simulink model "Simulator_Reduced"  (R2023a)
settings: Solver=ode4  StartTime=0.0  StopTime=Parameters.Simulink.sim_time_s  FixedStep=Parameters.Simulink.time_step_s  RelTol=1e-3
undefined symbols (not defined in the file): Parameters
libraries: eeGeneralControl x1
settings Model: Creator=thesa  LastModifiedBy=thesa
settings OptimizationCC: SimCompilerOptimization=on  AccelVerboseBuild=on
settings ModelReferenceCC: EnableParallelModelReferenceBuilds=on

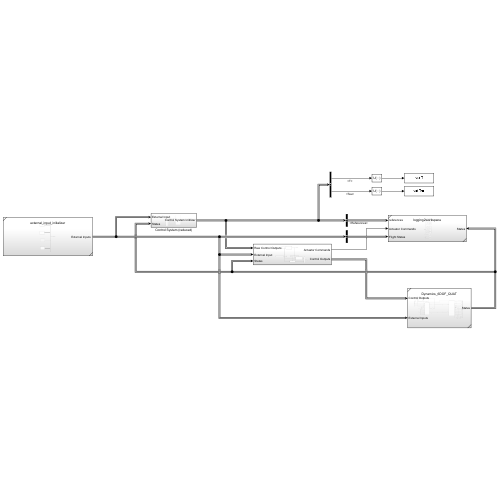
[thumbnail: Simulink's stored preview of the top-level diagram]
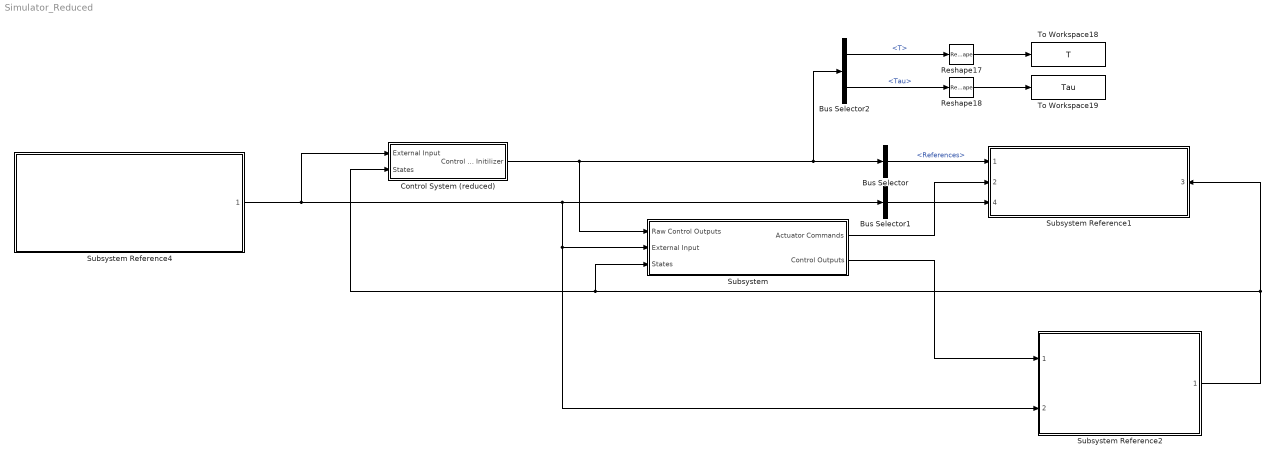
== system Simulator_Reduced ==
  Bus Selector : BusSelector  OutputSignals=References
  Bus Selector1 : BusSelector  OutputSignals=Pilot Input.ARMED,Pilot Input.FLIGHT_MODE  OutputAsBus=on
  Bus Selector2 : BusSelector  OutputSignals=Control Outputs.T,Control Outputs.Tau
  Control System (reduced) : Subsystem
  Reshape17 : Reshape
  Reshape18 : Reshape
  Subsystem : Subsystem
  Subsystem Reference1 : Subsystem  ReferencedSubsystem=logging2workspace
      settings: PortSchema="{\"entries\":[{\"content\":{\"sides\":[{\"content\":{\"connectorIds\":[\"In1\",\"In2\",\"In4\"]},\"type\":\"ConnectorPlacement.EquallySpacedRectSide\",\"uuid\":\"9edd3e15-5130-45dd-9916-21c08d031682\"},{\"content\":{\"connectorIds\":[\"In3\"],\"side\":\"RIGHT\"},\"type\":\"ConnectorPlacement.EquallySpacedRectSide\",\"uuid\":\"954423d3-db16-40ed-81b7-a6b5cde1e64c\"},{\"content\":{\"side\":\"TOP\"},\"type\":\"ConnectorPlacement.EquallySpacedRectSide\",\"uuid\":\"3251a3bf-10b0-45d6-866e-917fc661c50a\"}]},\"type\":\"ConnectorPlacement.EquallySpacedConnector\",\"uuid\":\"39e626d0-b0bd-4592-9fe5-df80528652ac\"}],\"packageUris\":[\"http://schema.mathworks.com/mf0/Connector/R2020b\"],\"version\":\"1.0\"}"
  Subsystem Reference2 : Subsystem  ReferencedSubsystem=Dynamics_6DOF_QUAT
  Subsystem Reference4 : Subsystem  ReferencedSubsystem=external_input_initializer
  To Workspace18 : ToWorkspace  VariableName=T  SampleTime=-1
  To Workspace19 : ToWorkspace  VariableName=Tau  SampleTime=-1
  wires:
  Subsystem Reference4/1 -> Bus Selector1/1, Subsystem Reference2/2, Subsystem/2(External Input), Control System (reduced)/1(External Input)
  Bus Selector/1 -> Subsystem Reference1/1  "<References>"
  Bus Selector1/1 -> Subsystem Reference1/4
  Control System (reduced)/1(Control System Initilizer) -> Subsystem/1(Raw Control Outputs), Bus Selector2/1, Bus Selector/1
  Reshape17/1 -> To Workspace18/1
  Reshape18/1 -> To Workspace19/1
  Bus Selector2/2 -> Reshape18/1  "<Tau>"
  Bus Selector2/1 -> Reshape17/1  "<T>"
  Subsystem/1(Actuator Commands) -> Subsystem Reference1/2
  Subsystem/2(Control Outputs) -> Subsystem Reference2/1
  Subsystem Reference2/1 -> Subsystem/3(States), Control System (reduced)/2(States), Subsystem Reference1/3

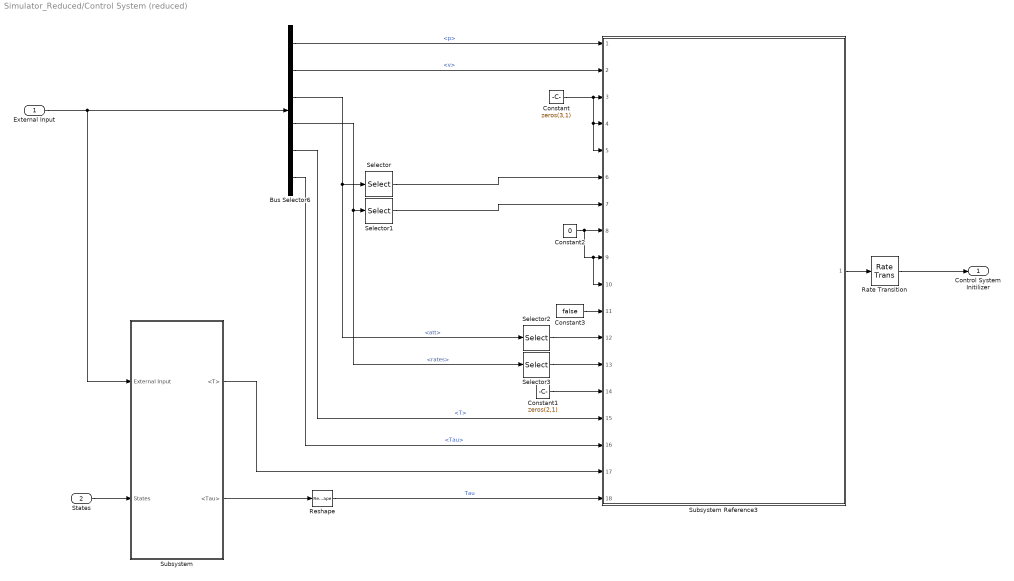
== system Simulator_Reduced/Control System (reduced) ==
  External Input : Inport
  States : Inport  Port=2
  Bus Selector6 : BusSelector  OutputSignals=Control Gains.K_matrix_control.ref.p,Control Gains.K_matrix_control.ref.v,Control Gains.K_matrix_control.ref.att,Control Gains.K_matrix_control.ref.rates,Control Gains.K_matrix_control.ref.T,Control Gains.K_matrix_control.ref.Tau
  Constant : Constant  Value=zeros(3,1)
  Constant1 : Constant  Value=zeros(2,1)
  Constant2 : Constant  Value=0
  Constant3 : Constant  Value=false
  Rate Transition : RateTransition  OutPortSampleTimeOpt=Inherit
  Reshape : Reshape  OutputDimensionality=Column vector (2-D)
  Selector : Selector  InputPortWidth=3  IndexOptions=Index vector (dialog)  Indices=[3]  OutputSizes=1
  Selector1 : Selector  InputPortWidth=3  IndexOptions=Index vector (dialog)  Indices=[3]  OutputSizes=1
  Selector2 : Selector  InputPortWidth=3  IndexOptions=Index vector (dialog)  Indices=[1,2]  OutputSizes=1
  Selector3 : Selector  InputPortWidth=3  IndexOptions=Index vector (dialog)  Indices=[1,2]  OutputSizes=1
  Subsystem : Subsystem
  Subsystem Reference3 : Subsystem  ReferencedSubsystem=control_initializer
  Control System Initilizer : Outport
  wires:
  Bus Selector6/3 -> Selector2/1, Selector/1  "<att>"
  External Input/1 -> Bus Selector6/1, Subsystem/1(External Input)
  Reshape/1 -> Subsystem Reference3/18  "Tau"
  Constant2/1 -> Subsystem Reference3/10, Subsystem Reference3/9, Subsystem Reference3/8
  Bus Selector6/4 -> Selector3/1, Selector1/1  "<rates>"
  Subsystem Reference3/1 -> Rate Transition/1
  Bus Selector6/1 -> Subsystem Reference3/1  "<p>"
  Bus Selector6/2 -> Subsystem Reference3/2  "<v>"
  Constant/1 -> Subsystem Reference3/5, Subsystem Reference3/4, Subsystem Reference3/3
  Selector/1 -> Subsystem Reference3/6
  Selector1/1 -> Subsystem Reference3/7
  Constant3/1 -> Subsystem Reference3/11
  Selector2/1 -> Subsystem Reference3/12
  Selector3/1 -> Subsystem Reference3/13
  Constant1/1 -> Subsystem Reference3/14
  Bus Selector6/5 -> Subsystem Reference3/15  "<T>"
  Bus Selector6/6 -> Subsystem Reference3/16  "<Tau>"
  Rate Transition/1 -> Control System Initilizer/1
  States/1 -> Subsystem/2(States)
  Subsystem/1(<T>) -> Subsystem Reference3/17
  Subsystem/2(<Tau>) -> Reshape/1

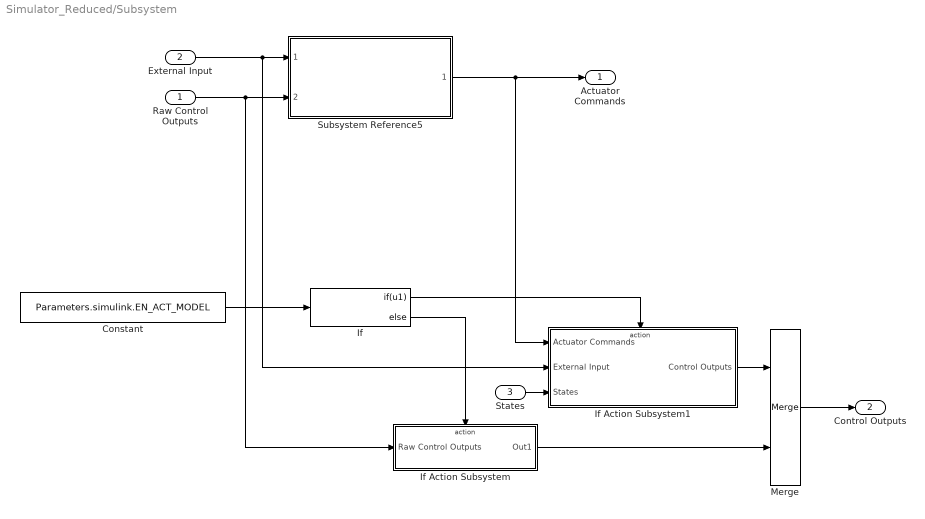
== system Simulator_Reduced/Subsystem ==
  Raw Control Outputs : Inport
  External Input : Inport  Port=2
  States : Inport  Port=3
  Constant : Constant  Value=Parameters.simulink.EN_ACT_MODEL
  If : If  IfExpression=u1
  If Action Subsystem : Subsystem  TreatAsAtomicUnit=on
  If Action Subsystem1 : Subsystem  TreatAsAtomicUnit=on
  Merge : Merge
  Subsystem Reference5 : Subsystem  ReferencedSubsystem=mixer
  Actuator Commands : Outport
  Control Outputs : Outport  Port=2
  wires:
  Subsystem Reference5/1 -> If Action Subsystem1/1(Actuator Commands), Actuator Commands/1
  Merge/1 -> Control Outputs/1
  External Input/1 -> If Action Subsystem1/2(External Input), Subsystem Reference5/1
  Raw Control Outputs/1 -> Subsystem Reference5/2, If Action Subsystem/1(Raw Control Outputs)
  If/1 -> If Action Subsystem1/Action
  If/2 -> If Action Subsystem/Action
  Constant/1 -> If/1
  If Action Subsystem1/1(Control Outputs) -> Merge/1
  If Action Subsystem/1(Out1) -> Merge/2
  States/1 -> If Action Subsystem1/3(States)

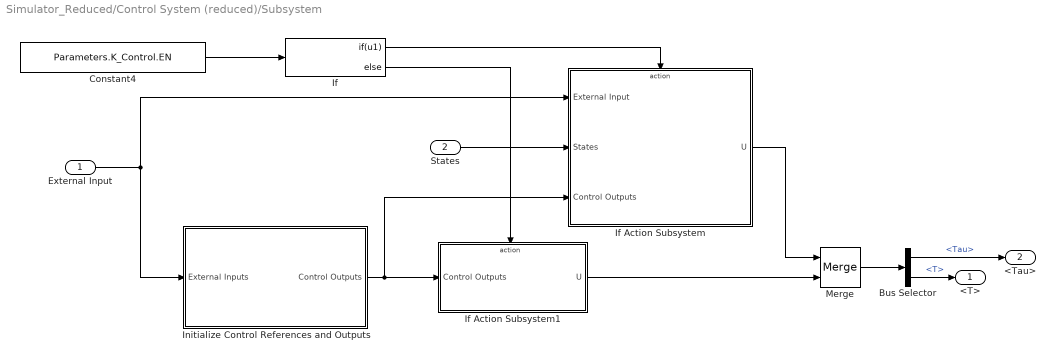
== system Simulator_Reduced/Control System (reduced)/Subsystem ==
  External Input : Inport
  States : Inport  Port=2
  Bus Selector : BusSelector  OutputSignals=Tau,T
  Constant4 : Constant  Value=Parameters.K_Control.EN
  If : If  IfExpression=u1
  If Action Subsystem : Subsystem  TreatAsAtomicUnit=on
  If Action Subsystem1 : Subsystem  TreatAsAtomicUnit=on
  Initialize Control References and Outputs : Subsystem
  Merge : Merge
  <T> : Outport
  <Tau> : Outport  Port=2
  wires:
  If/1 -> If Action Subsystem/Action
  Merge/1 -> Bus Selector/1
  If Action Subsystem/1(U) -> Merge/1
  If Action Subsystem1/1(U) -> Merge/2
  If/2 -> If Action Subsystem1/Action
  External Input/1 -> Initialize Control References and Outputs/1(External Inputs), If Action Subsystem/1(External Input)
  Constant4/1 -> If/1
  States/1 -> If Action Subsystem/2(States)
  Bus Selector/2 -> <T>/1  "<T>"
  Bus Selector/1 -> <Tau>/1  "<Tau>"
  Initialize Control References and Outputs/1(Control Outputs) -> If Action Subsystem/3(Control Outputs), If Action Subsystem1/1(Control Outputs)

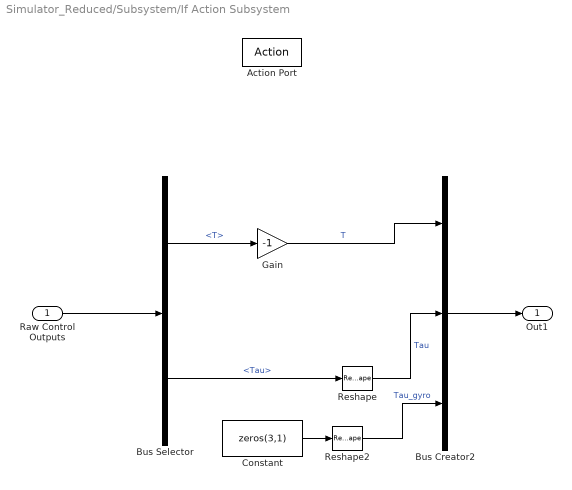
== system Simulator_Reduced/Subsystem/If Action Subsystem ==
  Raw Control Outputs : Inport
  Action Port : ActionPort  InitializeStates=reset  ActionPortLabel=else
  Bus Creator2 : BusCreator  Inputs=3
  Bus Selector : BusSelector  OutputSignals=Control Outputs.T,Control Outputs.Tau
  Constant : Constant  Value=zeros(3,1)
  Gain : Gain  Gain=-1
  Reshape : Reshape  OutputDimensionality=Column vector (2-D)
  Reshape2 : Reshape  OutputDimensionality=Column vector (2-D)
  Out1 : Outport
  wires:
  Bus Creator2/1 -> Out1/1
  Reshape/1 -> Bus Creator2/2  "Tau"
  Bus Selector/2 -> Reshape/1  "<Tau>"
  Bus Selector/1 -> Gain/1  "<T>"
  Raw Control Outputs/1 -> Bus Selector/1
  Gain/1 -> Bus Creator2/1  "T"
  Reshape2/1 -> Bus Creator2/3  "Tau_gyro"
  Constant/1 -> Reshape2/1

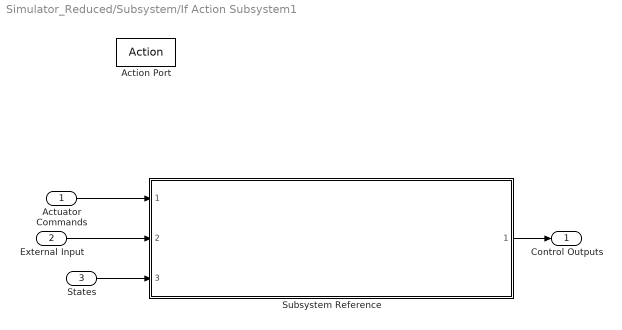
== system Simulator_Reduced/Subsystem/If Action Subsystem1 ==
  Actuator Commands : Inport
  External Input : Inport  Port=2
  States : Inport  Port=3
  Action Port : ActionPort  InitializeStates=reset  ActionPortLabel=if(u1)
  Subsystem Reference : Subsystem  ReferencedSubsystem=cmds2forces_map
  Control Outputs : Outport
  wires:
  Subsystem Reference/1 -> Control Outputs/1
  External Input/1 -> Subsystem Reference/2
  Actuator Commands/1 -> Subsystem Reference/1
  States/1 -> Subsystem Reference/3

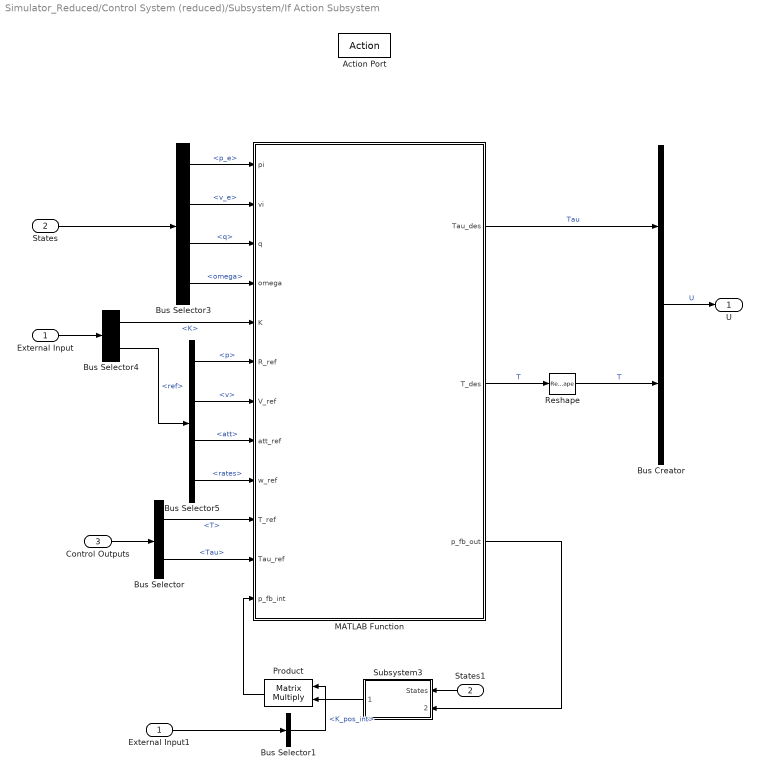
== system Simulator_Reduced/Control System (reduced)/Subsystem/If Action Subsystem ==
  External Input : Inport
  States : Inport  Port=2
  Control Outputs : Inport  Port=3
  Action Port : ActionPort  InitializeStates=reset  ActionPortLabel=if(u1)
  Bus Creator : BusCreator  Inputs=2
  Bus Selector : BusSelector  OutputSignals=T,Tau
  Bus Selector1 : BusSelector  OutputSignals=Control Gains.K_matrix_control.K_pos_int
  Bus Selector3 : BusSelector  OutputSignals=p_e,v_e,q,omega
  Bus Selector4 : BusSelector  OutputSignals=Control Gains.K_matrix_control.K,Control Gains.K_matrix_control.ref
  Bus Selector5 : BusSelector  OutputSignals=p,v,att,rates
  External Input1 : InportShadow
  MATLAB Function : MATLAB Function  TreatAsAtomicUnit=on
  Product : Product  Multiplication=Matrix(*)
  Reshape : Reshape  OutputDimensionality=Column vector (2-D)
  States1 : InportShadow  Port=2
  Subsystem3 : Subsystem
  U : Outport
  wires:
  Bus Selector5/4 -> MATLAB Function/9(w_ref)  "<rates>"
  MATLAB Function/2(T_des) -> Reshape/1  "T"
  Bus Selector4/2 -> Bus Selector5/1  "<ref>"
  Bus Selector3/2 -> MATLAB Function/2(vi)  "<v_e>"
  Bus Selector4/1 -> MATLAB Function/5(K)  "<K>"
  MATLAB Function/1(Tau_des) -> Bus Creator/1  "Tau"
  Bus Selector3/1 -> MATLAB Function/1(pi)  "<p_e>"
  Bus Selector3/3 -> MATLAB Function/3(q)  "<q>"
  States/1 -> Bus Selector3/1
  Bus Selector3/4 -> MATLAB Function/4(omega)  "<omega>"
  Bus Selector5/3 -> MATLAB Function/8(att_ref)  "<att>"
  Bus Selector5/2 -> MATLAB Function/7(V_ref)  "<v>"
  External Input/1 -> Bus Selector4/1
  Bus Selector5/1 -> MATLAB Function/6(R_ref)  "<p>"
  Reshape/1 -> Bus Creator/2  "T"
  Bus Creator/1 -> U/1  "U"
  External Input1/1 -> Bus Selector1/1
  Product/1 -> MATLAB Function/12(p_fb_int)
  Bus Selector1/1 -> Product/1  "<K_pos_int>"
  Subsystem3/1(p_fb_int) -> Product/2
  MATLAB Function/3(p_fb_out) -> Subsystem3/2(p_fb_out)
  States1/1 -> Subsystem3/1(States)
  Control Outputs/1 -> Bus Selector/1
  Bus Selector/1 -> MATLAB Function/10(T_ref)  "<T>"
  Bus Selector/2 -> MATLAB Function/11(Tau_ref)  "<Tau>"

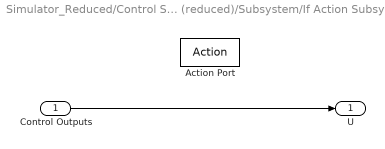
== system Simulator_Reduced/Control System (reduced)/Subsystem/If Action Subsystem1 ==
  Control Outputs : Inport
  Action Port : ActionPort  ActionPortLabel=else
  U : Outport
  wires:
  Control Outputs/1 -> U/1

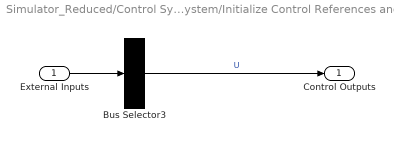
== system Simulator_Reduced/Control System (reduced)/Subsystem/Initialize Control References and Outputs ==
  External Inputs : Inport
  Bus Selector3 : BusSelector  OutputSignals=Control Gains.K_matrix_control.ref.Tau,Control Gains.K_matrix_control.ref.T  OutputAsBus=on
  Control Outputs : Outport
  wires:
  Bus Selector3/1 -> Control Outputs/1  "U"
  External Inputs/1 -> Bus Selector3/1

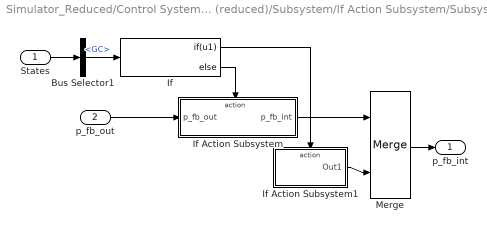
== system Simulator_Reduced/Control System (reduced)/Subsystem/If Action Subsystem/Subsystem3 ==
  States : Inport
  p_fb_out : Inport  Port=2
  Bus Selector1 : BusSelector  OutputSignals=GC
  If : If  IfExpression=u1
  If Action Subsystem : Subsystem  TreatAsAtomicUnit=on
  If Action Subsystem1 : Subsystem  TreatAsAtomicUnit=on
  Merge : Merge
  p_fb_int : Outport
  wires:
  Merge/1 -> p_fb_int/1
  If Action Subsystem1/1(Out1) -> Merge/2
  If Action Subsystem/1(p_fb_int) -> Merge/1
  If/2 -> If Action Subsystem/Action
  States/1 -> Bus Selector1/1
  p_fb_out/1 -> If Action Subsystem/1(p_fb_out)
  If/1 -> If Action Subsystem1/Action
  Bus Selector1/1 -> If/1  "<GC>"

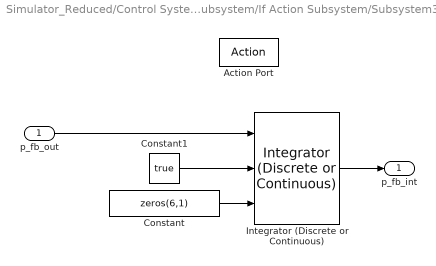
== system Simulator_Reduced/Control System (reduced)/Subsystem/If Action Subsystem/Subsystem3/If Action Subsystem ==
  p_fb_out : Inport
  Action Port : ActionPort  InitializeStates=reset  ActionPortLabel=else
  Constant : Constant  Value=zeros(6,1)
  Constant1 : Constant  Value=true
  Integrator (Discrete or Continuous) : eeGeneralControl/Integrator (Discrete or Continuous)  LabelModeActiveChoice=Discrete  ExternalReset=either  LimitType=Anti-windup  B=3  A=-3  Ts=-1
      settings: LibrarySourceBlock=|
      | ee_sl_lib/General Control/Integrator
      | (Discrete or Continuous)
  p_fb_int : Outport
  wires:
  p_fb_out/1 -> Integrator (Discrete or Continuous)/1
  Constant/1 -> Integrator (Discrete or Continuous)/3
  Integrator (Discrete or Continuous)/1 -> p_fb_int/1
  Constant1/1 -> Integrator (Discrete or Continuous)/2

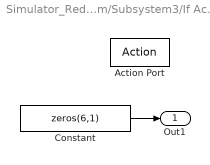
== system Simulator_Reduced/Control System (reduced)/Subsystem/If Action Subsystem/Subsystem3/If Action Subsystem1 ==
  Action Port : ActionPort  ActionPortLabel=if(u1)
  Constant : Constant  Value=zeros(6,1)
  Out1 : Outport
  wires:
  Constant/1 -> Out1/1

== matlab function Simulator_Reduced/Control System (reduced)/Subsystem/If Action Subsystem/MATLAB Function ==
  data: pi input; Tau_des output; vi input; q input; omega input; T_des output; K input; R_ref input; V_ref input; att_ref input; w_ref input; T_ref input; Tau_ref input; p_fb_int input; p_fb_out output
function [Tau_des, T_des, p_fb_out] = LQR_control(...
    pi, vi, q, omega, K,...
    R_ref, V_ref, att_ref, w_ref,...
    T_ref, Tau_ref, p_fb_int)
[Tau_des, T_des, p_fb_out] = LQR_control(...
    pi, vi, q, omega, K,...
    R_ref, V_ref, att_ref, w_ref,...
    T_ref, Tau_ref, p_fb_int);
end
